simulink model "Sampling_exp_5"  (R2021a)
settings: Solver=VariableStepAuto  StartTime=0.0  StopTime=10.0  RelTol=1e-3
libraries: dsparch4 x1
settings Model: Creator=Devraj Kashyap  LastModifiedBy=ritav

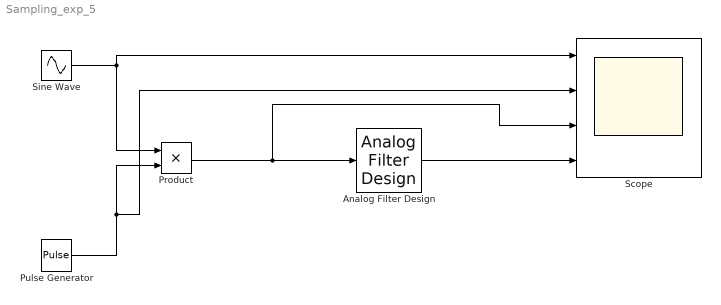
== system Sampling_exp_5 ==
  Analog Filter Design : dsparch4/Analog Filter Design  method=Butterworth  filttype=Lowpass  N=3  Wlo=2*pi*10  Whi=80  Rp=2  Rs=40
  Product : Product
  Pulse Generator : DiscretePulseGenerator  PulseType=Time based  Period=0.050  PulseWidth=5
  Scope : Scope  NumInputPorts=4
  Sine Wave : Sin  Amplitude=2  Frequency=2*pi*10  SampleTime=0.001
  wires:
  Sine Wave/1 -> Product/1, Scope/1
  Pulse Generator/1 -> Scope/2, Product/2
  Product/1 -> Scope/3, Analog Filter Design/1
  Analog Filter Design/1 -> Scope/4
